simulink model "pedcomp"  (R2023b)
settings: Solver=FixedStepAuto  StartTime=0.0  StopTime=10.0  FixedStep=50e-8  RelTol=1e-3
libraries: spspowerguiLib x1
settings Model: Creator=srini  LastModifiedBy=Vande

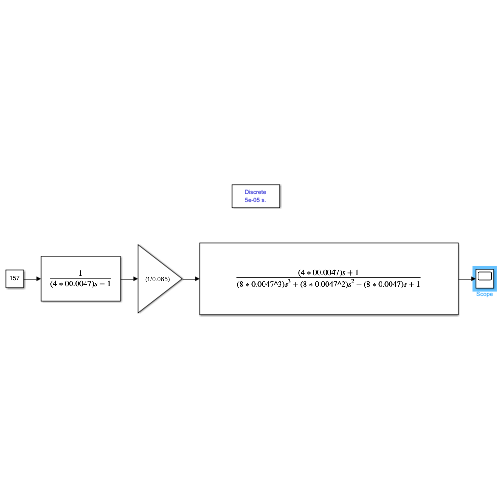
[thumbnail: Simulink's stored preview of the top-level diagram]
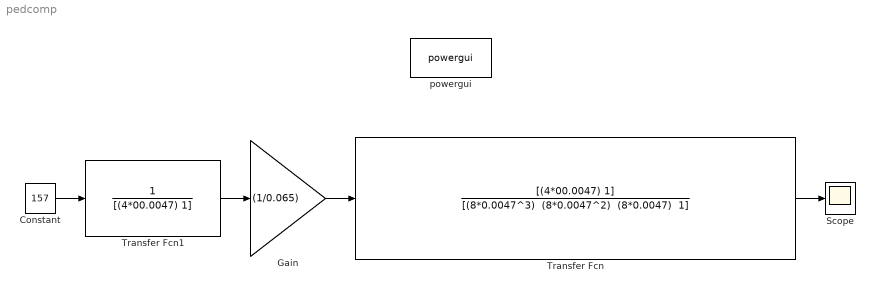
== system pedcomp ==
  Constant : Constant  Value=157
  Gain : Gain  Gain=(1/0.065)
  Scope : Scope
  Transfer Fcn : TransferFcn  Numerator=[(4*00.0047) 1]  Denominator="[(8*0.0047^3)  (8*0.0047^2)  (8*0.0047)  1]"
  Transfer Fcn1 : TransferFcn  Denominator=[(4*00.0047) 1]
  powergui : spspowerguiLib/powergui  Priority=1  SimulationMode=Discrete  SampleTime=50e-6  frequency=60  Iterations=50  frequencyindice=60  Pbase=100e6  ErrMax=1e-4  UnitsV=kV  UnitsW=MW  buscounter=0  FunctionMessages=off  echomessages=off  EnableUseOfTLC=off  CurrentSourceSwitches=off  DisableSnubberDevices=off  DisableRonSwitches=off  DisableVfSwitches=off  DisplayEquations=off  AutomaticDiscreteSolvers=off  SolverType=Tustin/Backward Euler (TBE)  Interpol=off  ExternalGateDelay=off  methode=off  Ts=100  x0status=blocks  SPID=on  SwTol=0  HookPort=off  NonlinearTolerance=1e-4  nMaxIteration=100  ContinueOnMaxIteration=off  RestoreLinks=warning  ResistiveCurrentMeasurement=off  Frange=[0:2:500]  Ylog=off  Xlog=on  ShowGrid=off  save=off  variable=ZData  structure=0  ZoomFFT=off  StartTime=0.0  cycles=1  DisplayStyle=1  fundamental=60  FreqAxis=off  MaxFrequency=1000  frequencyindicesteady=1  RmsSteady=1  display=off
  wires:
  Gain/1 -> Transfer Fcn/1
  Transfer Fcn1/1 -> Gain/1
  Transfer Fcn/1 -> Scope/1
  Constant/1 -> Transfer Fcn1/1
